simulink model "My_PWM"  (R2019b)
settings: Solver=ode23tb  StartTime=0.0  StopTime=10  RelTol=1e-3
libraries: simulink x1
settings Model: Creator=Sy2  LastModifiedBy=Sy2

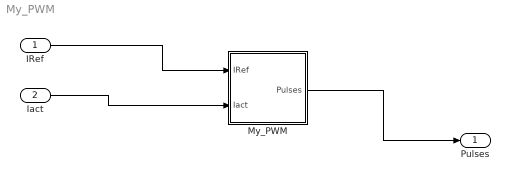
== system My_PWM ==
  "IRef " : Inport
  "Iact " : Inport  Port=2
  "My_PWM " : Subsystem
  "Pulses " : Outport
  wires:
  "IRef "/1 -> "My_PWM "/1("IRef ")
  "Iact "/1 -> "My_PWM "/2("Iact ")
  "My_PWM "/1("Pulses ") -> "Pulses "/1

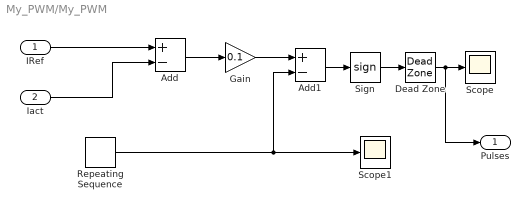
== system My_PWM/My_PWM  ==
  "IRef " : Inport
  "Iact " : Inport  Port=2
  Add : Sum  Inputs=+-
  Add1 : Sum  Inputs=+-
  Dead Zone : DeadZone  LowerValue=-10  UpperValue=0  SaturateOnIntegerOverflow=on
  Gain : Gain  Gain=0.1
  Repeating Sequence : simulink/Sources/Repeating Sequence  rep_seq_t=[0 1]  rep_seq_y=[0 1]
  Scope : Scope
  Scope1 : Scope
  Sign : Signum
  "Pulses " : Outport
  wires:
  Add/1 -> Gain/1
  "IRef "/1 -> Add/1
  Gain/1 -> Add1/1
  Repeating Sequence/1 -> Scope1/1, Add1/2
  Add1/1 -> Sign/1
  Dead Zone/1 -> "Pulses "/1, Scope/1
  Sign/1 -> Dead Zone/1
  "Iact "/1 -> Add/2
